simulink library "AEMS_Standard_Library"  (R2016b)
settings: Solver=ode45  StartTime=0.0  StopTime=10.0  RelTol=1e-3
undefined symbols (not defined in the file or in its folder): BkPY, carto, Cbx_extegr, Cbx_lpegrsys, Cbx_portegr, Cnx_bnk_nr_conf, Cnx_cyl_nr_conf, ConfigManagement, configuration_management, Cxx_dcm_io_tmr_end_xxxx, Cxx_dcm_rt_tmr_end, Cxx_DID_xxxx_IO_max, Cxx_DID_xxxx_IO_min, Cxx_egrhsofs, Cxx_vmaniegi, DEM_DEBOUNCE_FREEZE, DEM_DTR_CTL_INVISIBLE, DEM_DTR_CTL_NORMAL, Dem_DtrId2_XXX, Dem_DtrId3_XXX, Dem_DtrId4_XXX, Dem_DtrId5_XXX, Dem_DtrId6_XXX, Dem_DtrId7_XXX, Dem_DtrId8_XXX, Dem_DtrId9_XXX, Dem_DtrId_XXX, Dem_EnableConditionId2_XXX, Dem_EnableConditionId3_XXX, Dem_EnableConditionId4_XXX, Dem_EnableConditionId5_XXX, Dem_EnableConditionId6_XXX, Dem_EnableConditionId7_XXX, Dem_EnableConditionId8_XXX, Dem_EnableConditionId_XXX, Dem_EventId, Dem_EventId2_XXX, Dem_EventId3_XXX, Dem_EventId4_XXX, Dem_EventId5_XXX, Dem_EventId6_XXX, Dem_EventId7_XXX, Dem_EventId8_XXX, Dem_EventId9_XXX, Dem_EventId_Device_Faulttype, Dem_EventId_XXX, DEM_IUMPR_GENERAL_DENOMINATOR, DEM_OPCYC_IGNITION, Dem_RatioId2_XXX, Dem_RatioId3_XXX, Dem_RatioId4_XXX, Dem_RatioId5_XXX, Dem_RatioId6_XXX, Dem_RatioId7_XXX, Dem_RatioId8_XXX, Dem_RatioId_XXX, Dem_StorageConditionId2_XXX, Dem_StorageConditionId3_XXX, Dem_StorageConditionId4_XXX, Dem_StorageConditionId5_XXX ... (+65)
libraries: AEMS_Standard_Library x477, simulink x2
(part 2 of 39)

== system AEMS_Standard_Library/BIT_OPERATION ==
  AEMS_BITWISEAND : Subsystem  Tag=[LIB]  mask(AEMS_BITWISEAND){}
      mask help:
      | This block performs the BitwiseAND operation between the inputs "In","Mask",and the result is obtained at the outport "Out".
      |
      | NOTE:
      | Inputs must be positive integers, and the range should be 0 to ((2^32)-1).
      settings: AttributesFormatString=%<MaskType>
      mask Help:
      | eval('path_lib=fileparts(which(''AEMS_Standard_Library''));');
      | doc_path = [path_lib '\help\AEMS_BITWISEAND.pdf'];
      | eval('open(doc_path)')
      mask Display:
      | disp(['AEMS_BITWISEAND'])
      | port_label('input', 1, 'In');
      | port_label('input', 2, 'Mask');
      | port_label('output', 1, 'Out');
  AEMS_BITWISEOR : Subsystem  Tag=[LIB]  mask(AEMS_BITWISEOR){}
      mask help:
      | This block performs the BitwiseOR operation between the inputs "In","Mask",and the result is obtained at the outport "Out".
      |
      | NOTE:
      | Inputs must be positive integers, and the range should be 0 to ((2^32)-1).
      settings: AttributesFormatString=%<MaskType>
      mask Help:
      | eval('path_lib=fileparts(which(''AEMS_Standard_Library''));');
      | doc_path = [path_lib '\help\AEMS_BITWISEOR.pdf'];
      | eval('open(doc_path)')
      mask Display:
      | disp(['AEMS_BITWISEOR'])
      | port_label('input', 1, 'In');
      | port_label('input', 2, 'Mask');
      | port_label('output', 1, 'Out');
  AEMS_BITWISEXOR : Subsystem  Tag=[LIB]  mask(AEMS_BITWISEXOR){}
      mask help:
      | This block performs the BitwiseXOR operation between the inputs "In","Mask",and the result is obtained at the outport "Out".
      |
      | NOTE:
      | Inputs must be positive integers, and the range should be 0 to ((2^32)-1).
      settings: AttributesFormatString=%<MaskType>
      mask Help:
      | eval('path_lib=fileparts(which(''AEMS_Standard_Library''));');
      | doc_path = [path_lib '\help\AEMS_BITWISEXOR.pdf'];
      | eval('open(doc_path)')
      mask Display:
      | disp(['AEMS_BITWISEXOR'])
      | port_label('input', 1, 'In');
      | port_label('input', 2, 'Mask');
      | port_label('output', 1, 'Out');
  AEMS_BIT_GET : Subsystem  Tag=[LIB]  Description=|  mask(AEMS_BIT_GET){}
      | NOTE: The value of 'Bit_number' must be between 0 to 31.
      | The value of 'In' must be between 0 to (2^31)-1
      mask help:
      | This block extract the 'N'th Bit of the input 'In' and put it in the outport 'Bit_value'.
      | The value of 'N' is obtained from the inport 'Bit_number'.
      |
      | NOTE: The value of 'Bit_number' must be between 0 to 31. The value of 'In' must be between 0 to (2^31)-1.
      settings: AttributesFormatString=%<MaskType>
      mask Help:
      | eval('path_lib=fileparts(which(''AEMS_Standard_Library''));');
      | doc_path = [path_lib '\help\AEMS_BIT_GET.pdf'];
      | eval('open(doc_path)')
      mask Display:
      | disp('BitGet')
      | disp('\n\n LSB is Bit 0')
  AEMS_BIT_SET16 : Subsystem  Tag=[LIB]  mask(AEMS_BIT_SET16){}
      mask help:
      | The block performs the 16-bit binary to decimal conversion.
      | According to the values set for input bits(Bit1 to Bit16), 'Out' is the equivalent decimal value.
      | Note: All Input bits (Bit1 to Bit16) should be boolean
      settings: AttributesFormatString=%<MaskType>
      mask Help:
      | eval('path_lib=fileparts(which(''AEMS_Standard_Library''));');
      | doc_path = [path_lib '\help\AEMS_BIT_SET16.pdf'];
      | eval('open(doc_path)')
      mask Display: disp('AEMS_BIT_SET16')
  AEMS_BIT_SET32 : Subsystem  Tag=[LIB]  mask(AEMS_BIT_SET32){}
      mask help:
      | The block performs the 32-bit binary to decimal conversion.
      | According to the values set for input bits(Bit1 to Bit32), 'Out' is the equivalent decimal value.
      | Note: All Input bits (Bit1 to Bit32) should be boolean
      settings: AttributesFormatString=%<MaskType>
      mask Help:
      | eval('path_lib=fileparts(which(''AEMS_Standard_Library''));');
      | doc_path = [path_lib '\help\AEMS_BIT_SET32.pdf'];
      | eval('open(doc_path)')
      mask Display: disp('AEMS_BIT_SET32')
  AEMS_BIT_SET8 : Subsystem  Tag=[LIB]  mask(AEMS_BIT_SET8){}
      mask help:
      | The block performs the 8-bit binary to decimal conversion.
      | According to the values set for input bits(Bit1 to Bit8), 'out' is the equivalent decimal value.
      settings: AttributesFormatString=%<MaskType>
      mask Help:
      | eval('path_lib=fileparts(which(''AEMS_Standard_Library''));');
      | doc_path = [path_lib '\help\AEMS_BIT_SET8.pdf'];
      | eval('open(doc_path)')
      mask Display: disp('AEMS_BIT_SET8')
  AEMS_CONVERT_1BYTE_TO_2BYTE : Subsystem  Tag=[LIB]  mask(AEMS_CONVERT_1BYTE_TO_2BYTE){}
      mask help: Convert 1Byte to 2Byte.
      settings: AttributesFormatString=%<MaskType>
      mask Help:
      | eval('path_lib=fileparts(which(''AEMS_Standard_Library''));');
      | mskblk=get_param(gcbh,'MaskType');
      | doc_path = [path_lib '\help\',mskblk,'.pdf'];
      | eval('open(doc_path)');
      mask Display:
      | mask_disp = ['Convert\n1Byte to 2Byte'];
      | disp(mask_disp);
      | 
      | plot([5,5,5])
      | plot([6,6,6])
  AEMS_CONVERT_1BYTE_TO_8BIT : Subsystem  Tag=[LIB]  mask(AEMS_CONVERT_1BYTE_TO_8BIT){}
      mask help: Convert 1Byte to 8bit.
      settings: AttributesFormatString=%<MaskType>
      mask Help:
      | eval('path_lib=fileparts(which(''AEMS_Standard_Library''));');
      | mskblk=get_param(gcbh,'MaskType');
      | doc_path = [path_lib '\help\',mskblk,'.pdf'];
      | eval('open(doc_path)');
      mask Display:
      | mask_disp = ['Convert\n1Byte to 8bit\n\n\n'];
      | disp(mask_disp);
      | 
      | plot([5,5,5])
      | plot([6,6,6])
  AEMS_CONVERT_2BYTE_TO_1BYTE : Subsystem  Tag=[LIB]  mask(AEMS_CONVERT_2BYTE_TO_1BYTE){}
      mask help: Convert 2Byte to 1Byte
      settings: AttributesFormatString=%<MaskType>
      mask Help:
      | eval('path_lib=fileparts(which(''AEMS_Standard_Library''));');
      | mskblk=get_param(gcbh,'MaskType');
      | doc_path = [path_lib '\help\',mskblk,'.pdf'];
      | eval('open(doc_path)');
      mask Display:
      | mask_disp = ['Convert\n2Byte to 1Byte'];
      | disp(mask_disp);
      | 
      | plot([5,5,5])
      | plot([6,6,6])
  AEMS_CONVERT_8BIT_TO_1BYTE : Subsystem  Tag=[LIB]  mask(AEMS_CONVERT_8BIT_TO_1BYTE){}
      mask help: Convert 8bit to 1Byte.
      settings: AttributesFormatString=%<MaskType>
      mask Help:
      | eval('path_lib=fileparts(which(''AEMS_Standard_Library''));');
      | mskblk=get_param(gcbh,'MaskType');
      | doc_path = [path_lib '\help\',mskblk,'.pdf'];
      | eval('open(doc_path)');
      mask Display:
      | mask_disp = ['Convert\n8bit to 1Byte\n\n\n'];
      | disp(mask_disp);
      | 
      | plot([5,5,5])
      | plot([6,6,6])
  AEMS_CONVERT_TO_UNSIGNED_SI : Subsystem  Tag=[LIB]  Description=|  mask(AEMS_CONVERT_TO_UNSIGNED_SI){InputDataType=int16}
      | Converts a any integer to another one, of the same data size, containing the same stored value.
      | This operation can not do an overflow and thus is compliant with coding rules
      mask prompts: InputDataType "Input DataType"
      mask help:
      | Converts a any integer to another one, of the same data size, containing the same stored value.
      | This operation can not do an overflow and thus is compliant with coding rules
      mask init:
      | if(InputDataType == 1) %int8
      |     MS = 128;
      |     MABS = 127;
      |     u_inp_data = 'uint8';
      |     inp_data = 'int8';
      | elseif(InputDataType == 2) %int16
      |     MS = 32768;
      |     MABS = 32767;
      |     u_inp_data = 'uint16';
      |     inp_data = 'int16';
      | elseif(InputDataType == 3) %int32
      |     MS = 2147483648;
      |     MABS = 2147483647;
      |     u_inp_data = 'uint32';
      |     inp_data = 'int32';
      | end
      settings: AttributesFormatString="%<MaskType>\\nInput data type  = %<InputDataType>"
      mask Help:
      | eval('path_lib=fileparts(which(''AEMS_Standard_Library''));');
      | doc_path = [path_lib '\help\AEMS_CONVERT_TO_UNSIGNED_SI.pdf'];
      | eval('open(doc_path)')
      mask TypeOptions InputDataType: int8 | int16 | int32
      mask Display: disp('AEMS_CONVERT_TO_UNSIGNED_SI')
  AEMS_EXTRACT_BIT : Subsystem  Tag=[LIB]  Description=NOTE: The value of 'Number of bits' must be between 0 to 31.  mask(AEMS_EXTRACT_BIT){DataType=uint32, Value=Range starting with MSB, Range=[4,7], NB=28}
      mask prompts: DataType "Input DataType"; Value "Bits to extract:"; Range "Range of Bits"; NB "Number of bits"
      mask help:
      | AEMS_Extract_Bit Library block is used to extract the bits from the input In.
      | Based on the selection_mode and input data type the bits will be extracted.
      mask init:
      | extractBitBlock = gcb;
      | extractBitBlockH = gcbh;
      | 
      | %****************************************************************
      | 
      | Data_Value=get(extractBitBlockH,'Value');
      | if (strcmp(Data_Value,'Range of bits'))
      |     set_param(extractBitBlockH,'MaskVisibilities',{'on','on','on','off'})
      |     set(extractBitBlockH,'AttributesFormatString','%<MaskType>\nBits to extract = %<Value>\nInput data type  = %<DataType>\nRange of Bit: = %<Range>')
      | elseif (strcmp(Data_Value,'Range starting with MSB'))
      |     set_param(extractBitBlockH,'MaskVisibilities',{'on','on','off','on'})  
      |     set(extractBitBlockH,'AttributesFormatString','%<MaskType>\nBits to extract = %<Value>\nInput data type  = %<DataType>\nNumber of bits = %<NB>')
      | 
      | elseif (strcmp(Data_Value,'Range ending with LSB'))
      |     set_param(extractBitBlockH,'MaskVisibilities',{'on','on','off','on'})
      |     set(extractBitBlockH,'AttributesFormatString','%<MaskType>\nBits to extract = %<Value>\nInput data type  = %<DataType>\nNumber of bits = %<NB>')
      | 
      | else
      |     set_param(extractBitBlockH,'MaskVisibilities',{'on','on','off','off'})
      |     set(extractBitBlockH,'AttributesFormatString','%<MaskType>\nBits to extract = %<Value>\nInput data type  = %<DataType>')
      | 
      | end
      | 
      | %***************add or remove the conversion ********************
      | 
      | ConvertToUnsignedNoOverlowSS = [extractBitBlock,'/ConvertToUnsignedNoOverlow'];
      | 
      | 
      | if(DataType == 1 || DataType == 3 || DataType == 5) %unsigned
      |     try
      |         delete_line(extractBitBlock,'In/1','ConvertToUnsignedNoOverlow/1');
      |         delete_line(extractBitBlock,'ConvertToUnsignedNoOverlow/1', 'Chart/1');
      |         delete_block(ConvertToUnsignedNoOverlowSS);
      |     end
      |     try
      |         add_line(extractBitBlock,'In/1','Chart/1');
      |     end
      | elseif(DataType == 2 || DataType == 4 || DataType == 6) %signed
      |     try
      |         delete_line(extractBitBlock,'In/1','Chart/1');
      |     end
      |     try
      |         add_block('AEMS_Standard_Library/BIT_OPERATION/AEMS_CONVERT_TO_UNSIGNED_SI',ConvertToUnsignedNoOverlowSS);
      |         set_param(ConvertToUnsignedNoOverlowSS,'position',[70,146,285,184]);
      |         add_line(extractBitBlock,'In/1','ConvertToUnsignedNoOverlow/1');
      |         add_line(extractBitBlock,'ConvertToUnsignedNoOverlow/1','Chart/1');
      |     end
      |     try
      |         if(DataType == 2)
      |             set_param(ConvertToUnsignedNoOverlowSS,'InputDataType',0);
      |         elseif(DataType == 4)
      |             set_param(ConvertToUnsignedNoOverlowSS,'InputDataType',1);
      |         elseif(DataType == 6)
      |             set_param(ConvertToUnsignedNoOverlowSS,'InputDataType',2);
      |         end
      |     end
      | end
      | 
      | %****************************************************************
      | %************************uint8****int8***************************
      | if (DataType==1 || DataType == 2) 
      |     if (Value==1)           %  For Lower Half
      |         Max = 4;             
      |         LH = 2^(Max)-1;
      |         RH = 1;   
      |     elseif(Value==2)        %  For Upper Half
      |         Max = 8;
      |         LH = 2^(Max)-16;
      |         RH = 16;                %  Instead of right shift 4 bit for optimisation purpose divide the value by 2^4
      |     elseif(Value==3)        %  Range starting with most significant bit 
      |         RH = 2^(8-NB);
      |         LH = 255-(RH-1);        % value of selection of bits
      |     elseif(Value==4)        %  Range ending with least significant bit 
      |         LH = ((2^NB)- 1);
      |         RH = 1;
      |     else                    %  For Range of Bits 
      |         Min = Range(1);
      |         Max = Range(2);
      |         LH = (2^(Max+1)-1)-(2^Min-1);    % For Range of Bits
      |         RH = 2^Min;
      |     end
      |     u_inp_data = 'uint8';    
      | %****************************************************************
      | %************************uint16****int16*************************
      | elseif (DataType==3 || DataType==4)
      |     if (Value==1)           %  For Lower Half
      |         LH = 255;               % 0x00FF
      |         RH = 1;                 % 0x0001
      |     elseif(Value==2)        %  For Upper Half
      |         LH = 65280;             % 0xFF00
      |         RH = 256;               % 0x0100 %  Instead of right shift 4 bit for optimisation purpose divide the value by 2^8
      |     elseif(Value==3)        %  Range starting with most significant bit 
      |         RH = 2^(16-NB);         % 0xFF00 == 0d65280 (for 12 bits)
      |         LH = 65535-(RH-1);      % 0xFFFF - 0xFEFF = 0x0100 %  value of selection of bits
      |     elseif(Value==4)        %  Range ending with least significant bit 
      |         LH = ((2^NB)- 1);       % 0x0FFF (for 12 bits)
      |         RH = 1;                 % 0x0001
      |     else                    %  For Range of Bits 
      |         Min = Range(1);
      |         Max = Range(2);
      |         LH = (2^(Max+1)-1)-(2^Min-1);   
      |         RH = 2^Min;
      |     end
      |     u_inp_data = 'uint16';
      | %****************************************************************
      | %************************uint32*****int32************************
      | elseif (DataType==5 || DataType==6)
      |     if (Value==1)           %  For Lower Half
      |         LH=2^16-1;
      |         RH = 1;
      |     elseif(Value==2)        %  For Upper Half
      |         LH=2^32-65536;
      |         RH = 65536;              %  Instead of right shift 4 bit for optimisation purpose divide the value by 2^16 
      |     elseif(Value==3)        %  Range starting with most significant bit 
      |         RH = 2^(32-NB);          % 00100000
      |         LH = 4294967295 -(RH-1); % FFFFFFFF - 000FFFFF = FFF00000 value of selection of bits
      |     elseif(Value==4)        %  Range ending with least significant bit 
      |         LH = ((2^NB)- 1);
      |         RH = 1;
      |     else                    %  For Range of Bits 
      |         Min = Range(1);
      |         Max = Range(2);
      |         LH = (2^(Max+1)-1)-(2^Min-1); % For Range of Bits
      |         RH = 2^Min;
      | 
      |     end
      |     u_inp_data = 'uint32';
      | end
      | %****************************************************************
      settings: AttributesFormatString="%<MaskType>\\nBits to extract = %<Value>\\nInput data type  = %<DataType>\\nNumber of bits = %<NB>"  RTWSystemCode=Inline
      mask Help:
      | eval('path_lib=fileparts(which(''AEMS_Standard_Library''));');
      | doc_path = [path_lib '\help\AEMS_EXTRACT_BIT.pdf'];
      | eval('open(doc_path)')
      mask TypeOptions DataType: uint8 | int8 | uint16 | int16 | uint32 | int32
      mask TypeOptions Value: Lower Half | Upper Half | Range starting with MSB | Range ending with LSB | Range of bits
      mask Display: disp('AEMS_EXTRACT_BIT')

== system AEMS_Standard_Library/COM ==
  AEMS_FRAME_SUPERVISION : Subsystem  Tag=[LIB]  mask(AEMS_FRAME_SUPERVISION){}
      mask help:
      | This library block produces 4 supervisions information:
      |    1. Frame_Detected : Auto-detection Boolean of the ECU (TRUE - Supervised ECU frame is received)
      |    2. Status : Supervision ECU state. 3 possible states: Present, Absent, Validated Absent.
      |    3. Mon_Authorized : Boolean indicating if monitoring is enable.
      settings: AttributesFormatString=%<MaskType>
      mask Help:
      | eval('path_lib=fileparts(which(''AEMS_Standard_Library''));');
      | mskblk=get_param(gcbh,'MaskType');
      | doc_path = [path_lib '\help\',mskblk,'.pdf'];
      | eval('open(doc_path)');
  AEMS_REQUEST_COUNTER : Subsystem  Tag=[LIB]  mask(AEMS_REQUEST_COUNTER){Upper_Value=253}
      mask prompts: Upper_Value "Upper Limit"
      mask help:
      | This block is to output a repeating counter from Lower Limit to Upper_Limit with step one.
      | The counter increments at simulation start or whenever block is (placed in Runnable) triggered by an Event/Sched or a Boolean.
      |
      | Note:
      | Limits are to be Non-negative , Unsigned
      mask init:
      | ThisBlk=gcb;
      |  Bpath = [ThisBlk,'/Upper_Value'];
      |  set_param(Bpath,'Value',num2str(Upper_Value));
      |  
      |     if (Upper_Value <= 254)
      |       InpType = 'uint8';
      |       InpConTyp = 'uint8';
      |     elseif (Upper_Value == 255)
      |       InpType = 'uint16';
      |       InpConTyp = 'uint8';    
      |     elseif ((255 < Upper_Value) && (Upper_Value <= 65534))
      |       InpType = 'uint16';
      |       InpConTyp = 'uint16';
      |     elseif (Upper_Value == 65535)
      |       InpType = 'uint32';
      |       InpConTyp = 'uint16';    
      |     else
      |       InpType = 'uint32';
      |       InpConTyp = 'uint32';
      |     end
      settings: AttributesFormatString="%<MaskType> \\n Upper Limit  = %<Upper_Value>"  RTWSystemCode=Inline
      mask Help:
      | eval('path_lib=fileparts(which(''AEMS_Standard_Library''));');
      | mskblk=get_param(gcbh,'MaskType');
      | doc_path = [path_lib '\Help\',mskblk,'.pdf'];
      | eval('open(doc_path)');
      mask Display: port_label('output',1,'Request_Number')
  AEMS_REQUEST_COUNTER_SWITCH : Subsystem  Tag=[LIB]  mask(AEMS_REQUEST_COUNTER_SWITCH){Current_Value=1, Updated_Value=1}
      mask help: Output gets the value of "Current _Value" if the value of input "Request_Number" is not changed, else the Output takes the "Updated_Value".
      mask init:
      | ThisBlk =gcb;
      | Bpath = [ThisBlk,'/Current_Value'];
      | set_param(Bpath,'Value',num2str(Current_Value));
      | Bpath = [ThisBlk,'/Updated_Value'];
      | set_param(Bpath,'Value',num2str(Updated_Value));
      settings: RTWSystemCode=Inline
      settings: AttributesFormatString=|
      | %<MaskType>
      | Current_Value = %<Current_Value>\nUpdated_Value = %<Updated_Value>\n
      mask Help:
      | eval('path_lib=fileparts(which(''AEMS_Standard_Library''));');
      | mskblk=get_param(gcbh,'MaskType');
      | doc_path = [path_lib '\help\',mskblk,'.pdf'];
      | eval('open(doc_path)');

== system AEMS_Standard_Library/COUNTER ==
  AEMS_COUNTER : Subsystem  Tag=[LIB]  mask(AEMS_COUNTER){mMAX=1byte}
      mask prompts: mMAX "Max. count range :"
      mask help:
      | This block increments the counter value by 1 untill the count reaches the max limit.
      |
      | I/O
      |  start_flag
      |    1 : counter count up
      |    0 : counter hold
      |  clear_flag
      |    1 : counter clear
      |    0 : None
      |
      | count_value
      |    Counter value(up count)
      |
      | Reference to AUTOSAR specification:
      |            - AUTOSAR Service Name:  Efx_Counter_
      |            - Reference: SWS_Efx_00400
      mask init:
      | name=get_param(gcb,'MaskValueString');
      | switch mMAX
      |     case 1
      |         limit_value = 254;
      |         outDT = 'uint8';
      |     case 2
      |         limit_value = 65534;
      |         outDT = 'uint16';
      |     otherwise
      |         limit_value = 4294967294;
      |         outDT = 'uint32';
      | end
      | 
      | const_path = [gcb,'/Constant'];
      | for i=1:3
      |     set_param([const_path,num2str(i)],'OutDataTypeStr',outDT);
      | end
      settings: AttributesFormatString=%<MaskType>\nMax. count range = %<mMAX>
      mask Help:
      | eval('path_lib=fileparts(which(''AEMS_Standard_Library''));');
      | mskblk=get_param(gcbh,'MaskType');
      | doc_path = [path_lib '\help\',mskblk,'.pdf'];
      | eval('open(doc_path)');
      mask TypeOptions mMAX: 1byte | 2byte | 4byte
      mask Display: disp('AEMS_COUNTER');
